simulink model "light_control"  (R2021a)
settings: Solver=VariableStepAuto  StartTime=0.0  StopTime=10.0  RelTol=1e-3
settings Model: Creator=isacperez  LastModifiedBy=isacperez

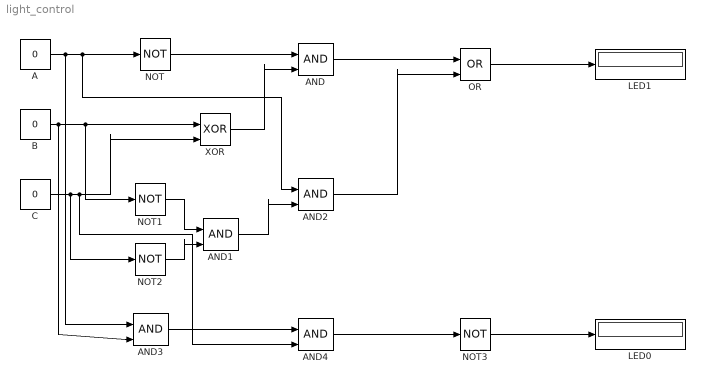
== system light_control ==
  A : Constant  Value=0
  AND{,1..4} (5 alike) : Logic  IconShape=distinctive  AllPortsSameDT=off  OutDataTypeStr=boolean
  B : Constant  Value=0
  C : Constant  Value=0
  LED0 : Display
  LED1 : Display
  NOT{,1..3} (4 alike) : Logic  Operator=NOT  IconShape=distinctive  AllPortsSameDT=off  OutDataTypeStr=boolean
  OR : Logic  Operator=OR  IconShape=distinctive  AllPortsSameDT=off  OutDataTypeStr=boolean
  XOR : Logic  Operator=XOR  IconShape=distinctive  AllPortsSameDT=off  OutDataTypeStr=boolean
  wires:
  A/1 -> AND3/1, AND2/1, NOT/1
  NOT/1 -> AND/1
  AND/1 -> OR/1
  OR/1 -> LED1/1
  B/1 -> AND3/2, NOT1/1, XOR/1
  XOR/1 -> AND/2
  AND2/1 -> OR/2
  AND1/1 -> AND2/2
  NOT1/1 -> AND1/1
  C/1 -> NOT2/1, AND4/2, XOR/2
  NOT2/1 -> AND1/2
  AND3/1 -> AND4/1
  AND4/1 -> NOT3/1
  NOT3/1 -> LED0/1
